simulink model "valid_rst_ramp"  (Simulink 7.6)
settings: Solver=ode45  StartTime=0.0  StopTime=1.0  RelTol=1e-3
undefined symbols (not defined in the file): DiscIntNeverNeededParam, Ks, R, S, T, tau, Te
settings Model: Creator=Jacques GANGLOFF  LastModifiedBy=jacques
settings OptimizationCC: InitFltsAndDblsToZero=on
settings DebuggingCC: StrictBusMsg=Warning

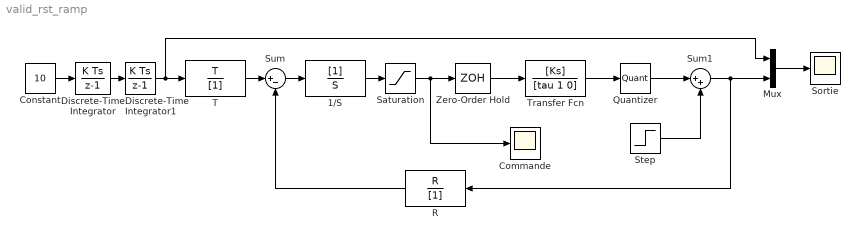
== system valid_rst_ramp ==
  1/S : DiscreteFilter  Denominator=S  SampleTime=Te
  Commande : Scope
  Constant : Constant  Value=10
  Discrete-Time Integrator : DiscreteIntegrator  SampleTime=Te  ICPrevOutput=DiscIntNeverNeededParam  ICPrevScaledInput=DiscIntNeverNeededParam
  Discrete-Time Integrator1 : DiscreteIntegrator  SampleTime=Te  ICPrevOutput=DiscIntNeverNeededParam  ICPrevScaledInput=DiscIntNeverNeededParam
  Mux : Mux  Inputs=2
  Quantizer : Quantizer  QuantizationInterval=1/180*pi
  R : DiscreteFilter  Numerator=R  Denominator=[1]  SampleTime=Te
  Saturation : Saturate  UpperLimit=100  LowerLimit=-100
  Sortie : Scope
  Step : Step  Time=0.5  After=0.5  SampleTime=0
  Sum : Sum  Inputs=|+-
  Sum1 : Sum  Inputs=|++
  T : DiscreteFilter  Numerator=T  Denominator=[1]  SampleTime=Te
  Transfer Fcn : TransferFcn  Numerator=[Ks]  Denominator=[tau 1 0]
  Zero-Order Hold : ZeroOrderHold  SampleTime=Te
  wires:
  Constant/1 -> Discrete-Time Integrator/1
  T/1 -> Sum/1
  Sum/1 -> 1/S/1
  1/S/1 -> Saturation/1
  Zero-Order Hold/1 -> Transfer Fcn/1
  Transfer Fcn/1 -> Quantizer/1
  R/1 -> Sum/2
  Mux/1 -> Sortie/1
  Quantizer/1 -> Sum1/1
  Sum1/1 -> Mux/2, R/1
  Step/1 -> Sum1/2
  Saturation/1 -> Zero-Order Hold/1, Commande/1
  Discrete-Time Integrator/1 -> Discrete-Time Integrator1/1
  Discrete-Time Integrator1/1 -> T/1, Mux/1
